simulink model "pid"  (R2023a)
settings: Solver=VariableStepAuto  StartTime=0.0  StopTime=10.0  RelTol=1e-3
settings Model: Creator=a2270170  LastModifiedBy=a2270170

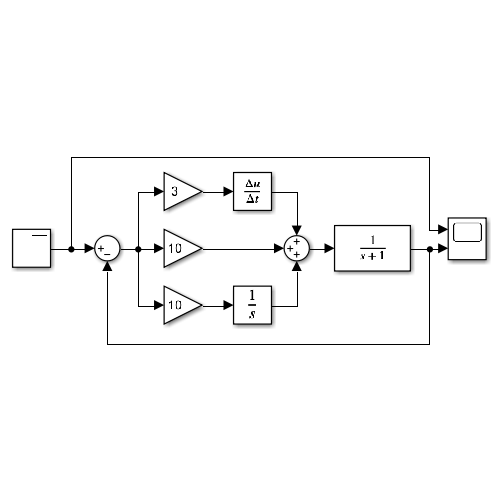
[thumbnail: Simulink's stored preview of the top-level diagram]
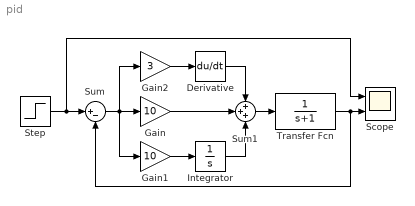
== system pid ==
  Derivative : Derivative
  Gain : Gain  Gain=10
  Gain1 : Gain  Gain=10
  Gain2 : Gain  Gain=3
  Integrator : Integrator
  Scope : Scope  NumInputPorts=2
  Step : Step  SampleTime=0
  Sum : Sum  Inputs=|+-
  Sum1 : Sum  Inputs=+++
  Transfer Fcn : TransferFcn  Denominator=[1 1]
  wires:
  Step/1 -> Sum/1, Scope/1
  Sum/1 -> Gain2/1, Gain1/1, Gain/1
  Transfer Fcn/1 -> Scope/2, Sum/2
  Sum1/1 -> Transfer Fcn/1
  Gain1/1 -> Integrator/1
  Gain2/1 -> Derivative/1
  Gain/1 -> Sum1/2
  Integrator/1 -> Sum1/3
  Derivative/1 -> Sum1/1
